simulink model "ported_ofdm_tx"  (R2017b)
settings: Solver=FixedStepDiscrete  StartTime=0.0  StopTime=10  RelTol=1e-3
libraries: commdigbbndam3 x16, hdlsllib x1, dspxfrm3 x1
settings Model: DataTypeOverride=Off  NumberOfSteps=100  Creator=jake  LastModifiedBy=root
settings DataIOCC: SaveOutput=off  SaveTime=off
settings OptimizationCC: BlockReduction=off  ConditionallyExecuteInputs=off  DefaultParameterBehavior=Inlined
settings DebuggingCC: AlgebraicLoopMsg=error  SingleTaskRateTransMsg=error  StrictBusMsg=ErrorOnBusTreatedAsVector
settings HardwareCC: ProdBitPerPointer=32  ProdBitPerSizeT=32  ProdBitPerPtrDiffT=32  ProdLargestAtomicFloat=None  ProdIntDivRoundTo=Undefined  ProdEndianess=Unspecified  ProdWordSize=32  ProdHWDeviceType=ASIC/FPGA->ASIC/FPGA  ProdEqTarget=off
settings CodeAppCC: StateflowObjectComments=on
settings GRTTargetCC: TargetLangStandard=C89/C90 (ANSI)

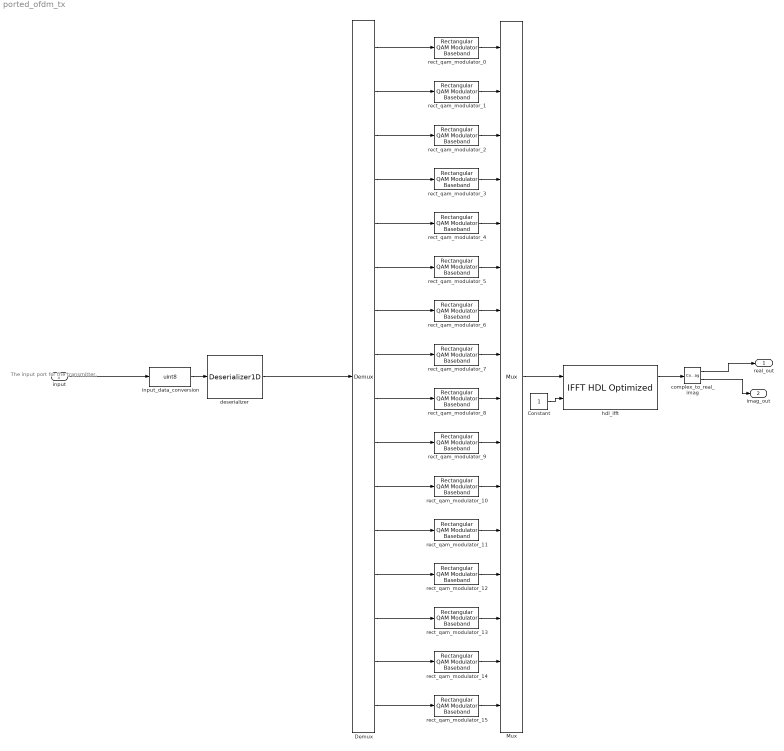
== system ported_ofdm_tx ==
  note: The input port for the transmitter.
  input : Inport
  Constant : Constant  OutDataTypeStr=boolean
  Demux : Demux  Outputs=16
  Mux : Mux  Inputs=16
  complex_to_real_imag : ComplexToRealImag
  deserializer : hdlsllib/HDL Operations/Deserializer1D  Ratio=16  IdleCycles=0  InitialCondition=0  startIn=off  validIn=off  validOut=off  inputDataDimensions=-1  inputSampleTime=-1  inputSignalType=auto
      settings: SourceProductName=HDL Coder  SourceProductBaseCode=HD
  hdl_ifft : dspxfrm3/IFFT HDL Optimized  FFTLength=16  Architecture=Streaming Radix 2^2  ComplexMultiplication=Use 3 multipliers and 5 adders  BitReversedOutput=on  BitReversedInput=off  Normalize=on  SimulateUsing=Code generation  RoundingMethod=Floor  ResetInputPort=off  StartOutputPort=off  EndOutputPort=off
      settings: SourceProductName=DSP System Toolbox  SourceProductBaseCode=DS
  input_data_conversion : DataTypeConversion  OutDataTypeStr=uint8
  rect_qam_modulator_{0..15} (16 alike) : commdigbbndam3/Rectangular QAM Modulator Baseband  M=16  InType=Integer  Enc=Gray  Mapping=[0:15]  PowType=Min. distance between symbols  MinDist=2  AvgPow=1  PeakPow=1  Ph=0  outDtype=Fixed-point  outWordLen=16  outUDDataType=sfix(16)  outFracLenMode=Best precision  outFracLen=15  outDataTypeStr=fixdt(1,16)  outLastDataTypeStr=fixdt(1,16)
  real_out : Outport  SignalName=ifft_real
  imag_out : Outport  Port=2  SignalName=ifft_imag
  wires:
  Demux/1 -> rect_qam_modulator_0/1
  Demux/2 -> rect_qam_modulator_1/1
  Demux/3 -> rect_qam_modulator_2/1
  Demux/4 -> rect_qam_modulator_3/1
  Demux/5 -> rect_qam_modulator_4/1
  Demux/6 -> rect_qam_modulator_5/1
  Demux/7 -> rect_qam_modulator_6/1
  Demux/8 -> rect_qam_modulator_7/1
  Demux/9 -> rect_qam_modulator_8/1
  Demux/10 -> rect_qam_modulator_9/1
  Demux/11 -> rect_qam_modulator_10/1
  Demux/12 -> rect_qam_modulator_11/1
  Demux/13 -> rect_qam_modulator_12/1
  Demux/14 -> rect_qam_modulator_13/1
  Demux/15 -> rect_qam_modulator_14/1
  Demux/16 -> rect_qam_modulator_15/1
  rect_qam_modulator_15/1 -> Mux/16
  rect_qam_modulator_14/1 -> Mux/15
  rect_qam_modulator_13/1 -> Mux/14
  rect_qam_modulator_12/1 -> Mux/13
  rect_qam_modulator_11/1 -> Mux/12
  rect_qam_modulator_10/1 -> Mux/11
  rect_qam_modulator_9/1 -> Mux/10
  rect_qam_modulator_8/1 -> Mux/9
  rect_qam_modulator_0/1 -> Mux/1
  rect_qam_modulator_1/1 -> Mux/2
  rect_qam_modulator_2/1 -> Mux/3
  rect_qam_modulator_3/1 -> Mux/4
  rect_qam_modulator_4/1 -> Mux/5
  rect_qam_modulator_5/1 -> Mux/6
  rect_qam_modulator_6/1 -> Mux/7
  rect_qam_modulator_7/1 -> Mux/8
  Mux/1 -> hdl_ifft/1
  hdl_ifft/1 -> complex_to_real_imag/1
  complex_to_real_imag/2 -> imag_out/1
  complex_to_real_imag/1 -> real_out/1
  Constant/1 -> hdl_ifft/2
  deserializer/1 -> Demux/1
  input_data_conversion/1 -> deserializer/1
  input/1 -> input_data_conversion/1
